simulink model "w2prob2"  (R2020a)
settings: Solver=VariableStepAuto  StartTime=0.0  StopTime=10.0  RelTol=1e-3
undefined symbols (not defined in the file): be, bv, Ie, Iv, muk, mus, R
settings Model: Creator=Anjali123  LastModifiedBy=Anjali123

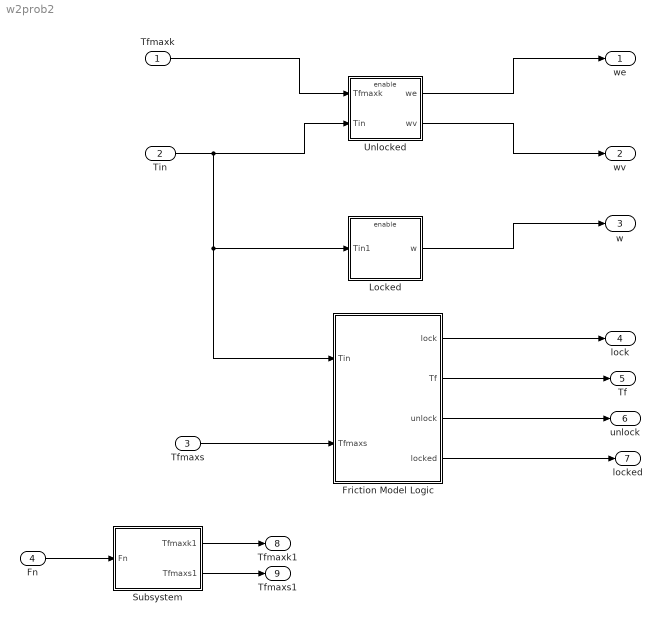
== system w2prob2 ==
  Tfmaxk : Inport
  Tin : Inport  Port=2
  Tfmaxs : Inport  Port=3
  Fn : Inport  Port=4
  Friction Model Logic : Subsystem
  Locked : Subsystem
  Subsystem : Subsystem
  Unlocked : Subsystem
  we : Outport  InitialOutput=0  VectorParamsAs1DForOutWhenUnconnected=off
  wv : Outport  Port=2  InitialOutput=0  VectorParamsAs1DForOutWhenUnconnected=off
  w : Outport  Port=3  InitialOutput=0  VectorParamsAs1DForOutWhenUnconnected=off
  lock : Outport  Port=4  InitialOutput=0  VectorParamsAs1DForOutWhenUnconnected=off
  Tf : Outport  Port=5  InitialOutput=0  VectorParamsAs1DForOutWhenUnconnected=off
  unlock : Outport  Port=6  InitialOutput=0  VectorParamsAs1DForOutWhenUnconnected=off
  locked : Outport  Port=7  InitialOutput=0  VectorParamsAs1DForOutWhenUnconnected=off
  Tfmaxk1 : Outport  Port=8  InitialOutput=0  VectorParamsAs1DForOutWhenUnconnected=off
  Tfmaxs1 : Outport  Port=9  InitialOutput=0  VectorParamsAs1DForOutWhenUnconnected=off
  wires:
  Tfmaxk/1 -> Unlocked/1(Tfmaxk)
  Unlocked/1(we) -> we/1
  Unlocked/2(wv) -> wv/1
  Locked/1(w) -> w/1
  Tin/1 -> Friction Model Logic/1(Tin), Locked/1(Tin1), Unlocked/2(Tin)
  Tfmaxs/1 -> Friction Model Logic/2(Tfmaxs)
  Friction Model Logic/1(lock) -> lock/1
  Friction Model Logic/2(Tf) -> Tf/1
  Friction Model Logic/3(unlock) -> unlock/1
  Friction Model Logic/4(locked) -> locked/1
  Fn/1 -> Subsystem/1(Fn)
  Subsystem/1(Tfmaxk1) -> Tfmaxk1/1
  Subsystem/2(Tfmaxs1) -> Tfmaxs1/1

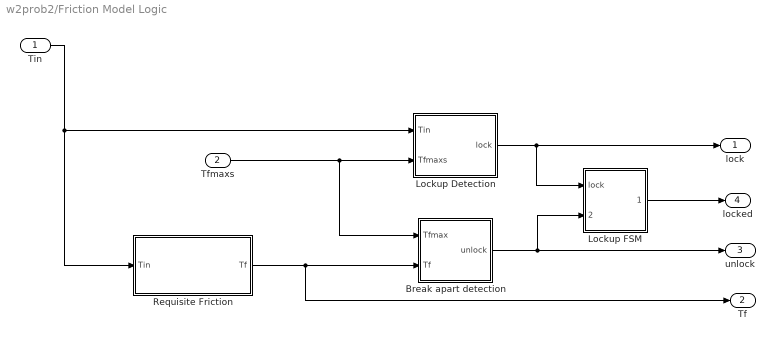
== system w2prob2/Friction Model Logic ==
  Tin : Inport
  Tfmaxs : Inport  Port=2
  Break apart detection : Subsystem
  Lockup Detection : Subsystem
  Lockup FSM : Subsystem
  Requisite Friction : Subsystem
  lock : Outport  InitialOutput=0  VectorParamsAs1DForOutWhenUnconnected=off
  Tf : Outport  Port=2  InitialOutput=0  VectorParamsAs1DForOutWhenUnconnected=off
  unlock : Outport  Port=3  InitialOutput=0  VectorParamsAs1DForOutWhenUnconnected=off
  locked : Outport  Port=4  InitialOutput=0  VectorParamsAs1DForOutWhenUnconnected=off
  wires:
  Break apart detection/1(unlock) -> unlock/1, Lockup FSM/2(unlock)
  Lockup Detection/1(lock) -> lock/1, Lockup FSM/1(lock)
  Tin/1 -> Requisite Friction/1(Tin), Lockup Detection/1(Tin)
  Requisite Friction/1(Tf) -> Tf/1, Break apart detection/2(Tf)
  Tfmaxs/1 -> Break apart detection/1(Tfmax), Lockup Detection/2(Tfmaxs)
  Lockup FSM/1(locked) -> locked/1

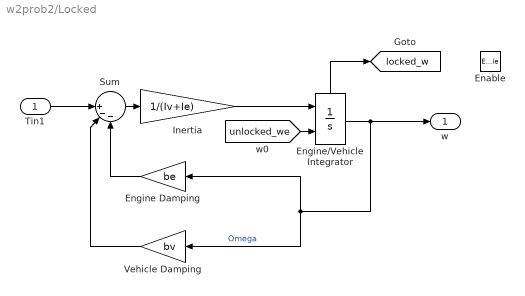
== system w2prob2/Locked ==
  Tin1 : Inport
  Enable : EnablePort
  Engine Damping : Gain  Gain=be  SaturateOnIntegerOverflow=on  OutDataTypeStr=Inherit: Same as input  ParamDataTypeStr=Inherit: Same as input
  Engine/Vehicle Integrator : Integrator  InitialConditionSource=external  ShowStatePort=on
  Inertia : Gain  Gain=1/(Iv+Ie)  SaturateOnIntegerOverflow=on  OutDataTypeStr=Inherit: Same as input  ParamDataTypeStr=Inherit: Same as input
  Sum : Sum  Inputs=||+--  InputSameDT=on  SaturateOnIntegerOverflow=on  OutDataTypeStr=Inherit: Same as first input
  Vehicle Damping : Gain  Gain=bv  SaturateOnIntegerOverflow=on  OutDataTypeStr=Inherit: Same as input  ParamDataTypeStr=Inherit: Same as input
  w : Outport  InitialOutput=0  VectorParamsAs1DForOutWhenUnconnected=off
  tag scope: locked_w=global
  wires:
  Engine/Vehicle Integrator/1 -> w/1, Engine Damping/1, Vehicle Damping/1  "Omega"
  Vehicle Damping/1 -> Sum/2
  Inertia/1 -> Engine/Vehicle Integrator/1
  Sum/1 -> Inertia/1
  Engine Damping/1 -> Sum/3
  Engine/Vehicle Integrator/State -> [locked_w]
  Tin1/1 -> Sum/1
  [unlocked_we] -> Engine/Vehicle Integrator/2

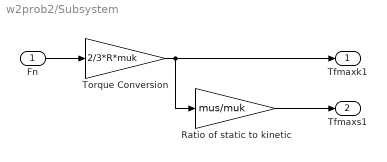
== system w2prob2/Subsystem ==
  Fn : Inport
  Ratio of static to kinetic : Gain  Gain=mus/muk  SaturateOnIntegerOverflow=on  OutDataTypeStr=Inherit: Same as input  ParamDataTypeStr=Inherit: Same as input
  Torque Conversion : Gain  Gain=2/3*R*muk  SaturateOnIntegerOverflow=on  OutDataTypeStr=Inherit: Same as input  ParamDataTypeStr=Inherit: Same as input
  Tfmaxk1 : Outport  InitialOutput=0  VectorParamsAs1DForOutWhenUnconnected=off
  Tfmaxs1 : Outport  Port=2  InitialOutput=0  VectorParamsAs1DForOutWhenUnconnected=off
  wires:
  Fn/1 -> Torque Conversion/1
  Torque Conversion/1 -> Tfmaxk1/1, Ratio of static to kinetic/1
  Ratio of static to kinetic/1 -> Tfmaxs1/1

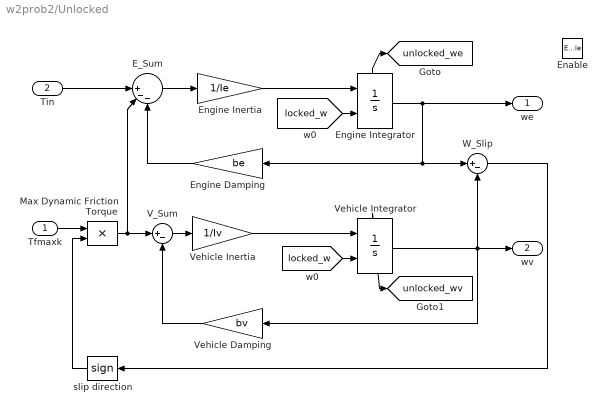
== system w2prob2/Unlocked ==
  Tfmaxk : Inport
  Tin : Inport  Port=2
  Enable : EnablePort
  E_Sum : Sum  Inputs=||+--  InputSameDT=on  SaturateOnIntegerOverflow=on  OutDataTypeStr=Inherit: Same as first input
  Engine Damping : Gain  Gain=be  SaturateOnIntegerOverflow=on  OutDataTypeStr=Inherit: Same as input  ParamDataTypeStr=Inherit: Same as input
  Engine Inertia : Gain  Gain=1/Ie  SaturateOnIntegerOverflow=on  OutDataTypeStr=Inherit: Same as input  ParamDataTypeStr=Inherit: Same as input
  Engine Integrator : Integrator  InitialConditionSource=external  ShowStatePort=on
  Max Dynamic Friction Torque : Product  InputSameDT=on  RndMeth=Zero  SaturateOnIntegerOverflow=on  OutDataTypeStr=Inherit: Same as first input
  V_Sum : Sum  Inputs=|+-  InputSameDT=on  SaturateOnIntegerOverflow=on  OutDataTypeStr=Inherit: Same as first input
  Vehicle Damping : Gain  Gain=bv  SaturateOnIntegerOverflow=on  OutDataTypeStr=Inherit: Same as input  ParamDataTypeStr=Inherit: Same as input
  Vehicle Inertia : Gain  Gain=1/Iv  SaturateOnIntegerOverflow=on  OutDataTypeStr=Inherit: Same as input  ParamDataTypeStr=Inherit: Same as input
  Vehicle Integrator : Integrator  InitialConditionSource=external  ShowStatePort=on
  W_Slip : Sum  Inputs=|+-  InputSameDT=on  SaturateOnIntegerOverflow=on  OutDataTypeStr=Inherit: Same as first input
  slip direction : Signum
  we : Outport  InitialOutput=0  VectorParamsAs1DForOutWhenUnconnected=off
  wv : Outport  Port=2  InitialOutput=0  VectorParamsAs1DForOutWhenUnconnected=off
  tag scope: unlocked_we=global, unlocked_wv=global
  wires:
  Vehicle Integrator/State -> [unlocked_wv]
  Vehicle Integrator/1 -> wv/1, W_Slip/2, Vehicle Damping/1
  Vehicle Inertia/1 -> Vehicle Integrator/1
  Tin/1 -> E_Sum/1
  W_Slip/1 -> slip direction/1
  Vehicle Damping/1 -> V_Sum/2
  [locked_w] -> Vehicle Integrator/2
  V_Sum/1 -> Vehicle Inertia/1
  Engine Inertia/1 -> Engine Integrator/1
  E_Sum/1 -> Engine Inertia/1
  Engine Integrator/State -> [unlocked_we]
  Tfmaxk/1 -> Max Dynamic Friction Torque/1
  slip direction/1 -> Max Dynamic Friction Torque/2
  Max Dynamic Friction Torque/1 -> V_Sum/1, E_Sum/2
  Engine Integrator/1 -> we/1, Engine Damping/1, W_Slip/1
  [locked_w] -> Engine Integrator/2
  Engine Damping/1 -> E_Sum/3

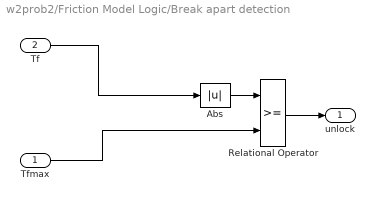
== system w2prob2/Friction Model Logic/Break apart detection ==
  Tfmax : Inport
  Tf : Inport  Port=2
  Abs : Abs  SaturateOnIntegerOverflow=on
  Relational Operator : RelationalOperator  OutDataTypeStr=boolean  RndMeth=Nearest  InputSameDT=on
  unlock : Outport  InitialOutput=0  VectorParamsAs1DForOutWhenUnconnected=off
  wires:
  Abs/1 -> Relational Operator/1
  Tf/1 -> Abs/1
  Tfmax/1 -> Relational Operator/2
  Relational Operator/1 -> unlock/1

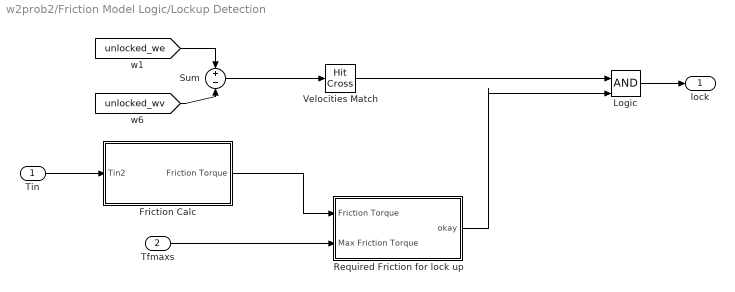
== system w2prob2/Friction Model Logic/Lockup Detection ==
  Tin : Inport
  Tfmaxs : Inport  Port=2
  Friction Calc : Subsystem
  Logic : Logic  IconShape=distinctive  OutDataTypeStr=boolean
  Required Friction for lock up : Subsystem
  Sum : Sum  Inputs=+-  InputSameDT=on  SaturateOnIntegerOverflow=on  OutDataTypeStr=Inherit: Same as first input
  Velocities Match : HitCross
  lock : Outport  InitialOutput=0  VectorParamsAs1DForOutWhenUnconnected=off
  wires:
  Tin/1 -> Friction Calc/1(Tin2)
  Required Friction for lock up/1(okay) -> Logic/2
  Friction Calc/1(Friction Torque) -> Required Friction for lock up/1(Friction Torque)
  [unlocked_we] -> Sum/1
  Tfmaxs/1 -> Required Friction for lock up/2(Max Friction Torque)
  [unlocked_wv] -> Sum/2
  Logic/1 -> lock/1
  Sum/1 -> Velocities Match/1
  Velocities Match/1 -> Logic/1

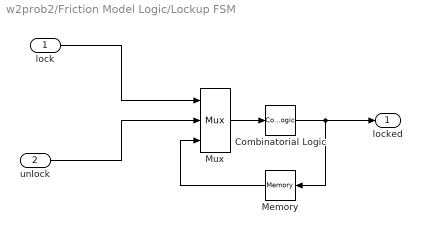
== system w2prob2/Friction Model Logic/Lockup FSM ==
  lock : Inport
  unlock : Inport  Port=2
  Combinatorial Logic : CombinatorialLogic  TruthTable=[0;1;0;0;1;1;1;0]
  Memory : Memory
  Mux : Mux  Inputs=3
  locked : Outport  InitialOutput=0  VectorParamsAs1DForOutWhenUnconnected=off
  wires:
  Mux/1 -> Combinatorial Logic/1
  Combinatorial Logic/1 -> locked/1, Memory/1
  lock/1 -> Mux/1
  Memory/1 -> Mux/3
  unlock/1 -> Mux/2

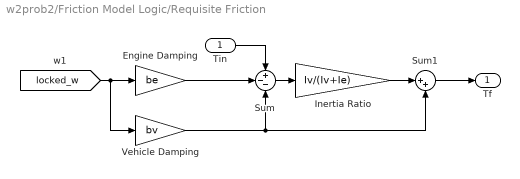
== system w2prob2/Friction Model Logic/Requisite Friction ==
  Tin : Inport
  Engine Damping : Gain  Gain=be  SaturateOnIntegerOverflow=on  OutDataTypeStr=Inherit: Same as input  ParamDataTypeStr=Inherit: Same as input
  Inertia Ratio : Gain  Gain=Iv/(Iv+Ie)  SaturateOnIntegerOverflow=on  OutDataTypeStr=Inherit: Same as input  ParamDataTypeStr=Inherit: Same as input
  Sum : Sum  Inputs=+--  InputSameDT=on  SaturateOnIntegerOverflow=on  OutDataTypeStr=Inherit: Same as first input
  Sum1 : Sum  Inputs=|++  InputSameDT=on  SaturateOnIntegerOverflow=on  OutDataTypeStr=Inherit: Same as first input
  Vehicle Damping : Gain  Gain=bv  SaturateOnIntegerOverflow=on  OutDataTypeStr=Inherit: Same as input  ParamDataTypeStr=Inherit: Same as input
  Tf : Outport  InitialOutput=0  VectorParamsAs1DForOutWhenUnconnected=off
  wires:
  Inertia Ratio/1 -> Sum1/1
  Vehicle Damping/1 -> Sum/3, Sum1/2
  Sum/1 -> Inertia Ratio/1
  Engine Damping/1 -> Sum/2
  Sum1/1 -> Tf/1
  Tin/1 -> Sum/1
  [locked_w] -> Vehicle Damping/1, Engine Damping/1

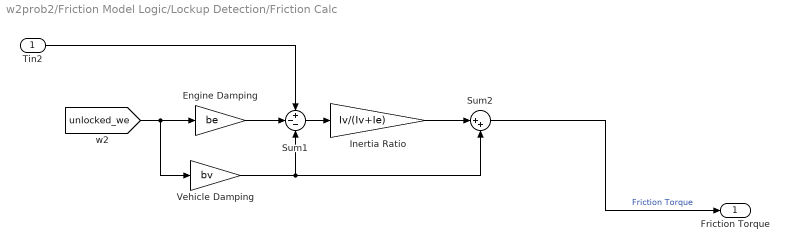
== system w2prob2/Friction Model Logic/Lockup Detection/Friction Calc ==
  Tin2 : Inport
  Engine Damping : Gain  Gain=be  SaturateOnIntegerOverflow=on  OutDataTypeStr=Inherit: Same as input  ParamDataTypeStr=Inherit: Same as input
  Inertia Ratio : Gain  Gain=Iv/(Iv+Ie)  SaturateOnIntegerOverflow=on  OutDataTypeStr=Inherit: Same as input  ParamDataTypeStr=Inherit: Same as input
  Sum1 : Sum  Inputs=+--  InputSameDT=on  SaturateOnIntegerOverflow=on  OutDataTypeStr=Inherit: Same as first input
  Sum2 : Sum  Inputs=|++  InputSameDT=on  SaturateOnIntegerOverflow=on  OutDataTypeStr=Inherit: Same as first input
  Vehicle Damping : Gain  Gain=bv  SaturateOnIntegerOverflow=on  OutDataTypeStr=Inherit: Same as input  ParamDataTypeStr=Inherit: Same as input
  Friction Torque : Outport
  wires:
  Sum1/1 -> Inertia Ratio/1
  Sum2/1 -> Friction Torque/1  "Friction Torque"
  Tin2/1 -> Sum1/1
  Inertia Ratio/1 -> Sum2/1
  Vehicle Damping/1 -> Sum2/2, Sum1/3
  [unlocked_we] -> Engine Damping/1, Vehicle Damping/1
  Engine Damping/1 -> Sum1/2

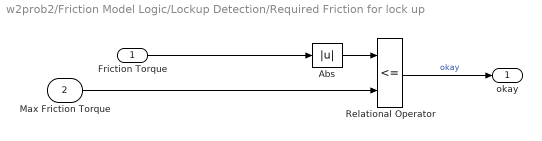
== system w2prob2/Friction Model Logic/Lockup Detection/Required Friction for lock up ==
  Friction Torque : Inport
  Max Friction Torque : Inport  Port=2
  Abs : Abs  SaturateOnIntegerOverflow=on
  Relational Operator : RelationalOperator  Operator=<=  OutDataTypeStr=boolean  RndMeth=Nearest  InputSameDT=on
  okay : Outport
  wires:
  Max Friction Torque/1 -> Relational Operator/2
  Abs/1 -> Relational Operator/1
  Relational Operator/1 -> okay/1  "okay"
  Friction Torque/1 -> Abs/1
